simulink model "an_ch"  (Simulink 3.00)
settings: Solver=ode45  StartTime=0.0  StopTime=20  MaxStep=.01  RelTol=1e-3  AbsTol=1e-3
values from neighbouring files (symbols this model uses):
  den = 1    [ASS1_SIS.M]    (also in ASS_APPR.M; ASS_SIS.M; MYFBODE.M = b; MYNYQ.M = b)
  den_c = 1    [ASS1_SIS.M]    (also in ASS2_CN.M; ASS_C.M; ASS_SIS.M)
  num = 0    [ASS1_SIS.M]    (also in ASS_SIS.M; MYFBODE.M = a; MYNYQ.M = a; nyquistnew.m = a)
  num_c = 0    [ASS1_SIS.M]    (also in ASS2_CN.M; ASS_C.M; ASS_SIS.M)
  T = 0    [ASS1_SIS.M]    (also in ASS_APPR.M = 0; end; ASS_SIS.M; MYFBODE.M = rit)
undefined symbols (not defined in the file or in its folder): sfunyst
settings Model: SaveTime=off  SaveOutput=off  LastModifiedBy=Administrator

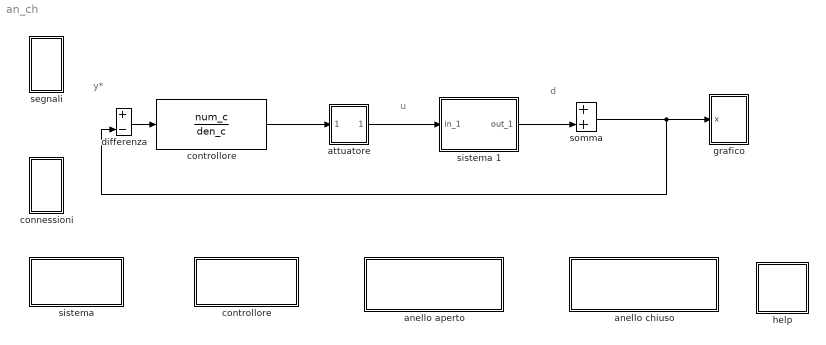
== system an_ch ==
  note: u
  note: d
  note: y*
  anello aperto : Subsystem
      mask Display: disp('analisi\n in anello aperto')
  anello chiuso : Subsystem
      mask Display: disp('analisi\n in anello chiuso')
  attuatore : Subsystem  mask{upperlimit=inf, lowerlimit=-inf}
      mask prompts: upperlimit "limite superiore"; lowerlimit "limite inferiore"
      mask Display: disp('A')
  connessioni : Subsystem
  controllore : Subsystem
      mask Display: disp('controllore')
  "controllore " : TransferFcn  Numerator=num_c  Denominator=den_c
      settings: OpenFcn=blocca
      mask Display: disp('controllore')
  differenza : Sum  Inputs=+-  SaturateOnIntegerOverflow=on
  grafico : Subsystem  mask(Storage scope.){@1=2, @2=-10, @3=10, @4=2000, @5='b-/r-/c-./w:/m*/ro/b+'}
      mask prompts: @1 "Initial Time Range:"; @2 "Initial y-min:"; @3 "Initial y-max:"; @4 "Storage pts.:"; @5 "Line type (rgbw-.:xo):"
      mask help:
      | Storage scope using MATLAB graph window.
      | Enter plotting ranges and line type.
      mask init:
      | npts = @4; color = @5; ax = [0, @1, @2, @3]; dt=-1;
      mask Help: This block uses a MATLAB figure window to plot the input signal.  The graph limits are automatically scaled to the min and max values of the signal stored in the scope's signal buffer.  Line type must be in quotes.  See the M-file sfunyst.m.
      mask Display: plot(0,0,100,100,[83,76,63,52,42,38,28,16,11,84,11,11,11,90,90,11],[75,58,47,54,72,80,84,74,65,65,65,90,40,40,90,90])
  help : Subsystem
      mask Display: disp('?')
  segnali : Subsystem
  sistema : Subsystem
      mask Display: disp('sistema')
  sistema 1 : Subsystem
      settings: OpenFcn=blocca
      mask Display: disp('sistema')
  "somma " : Sum  Inputs=++  SaturateOnIntegerOverflow=on
  wires:
  sistema 1/1(out_1) -> "somma "/2
  differenza/1 -> "controllore "/1
  "controllore "/1 -> attuatore/1(In1)
  attuatore/1(Out1) -> sistema 1/1(in_1)
  "somma "/1 -> grafico/1(x), differenza/2

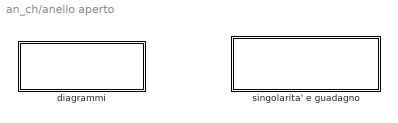
== system an_ch/anello aperto ==
  diagrammi : Subsystem
      mask Display: disp('diagrammi\n  \n (Bode e Nyquist)')
  singolarita' e guadagno : Subsystem
      settings: OpenFcn=sing_tot
      mask Type: singolarita' della f.d.t.
      mask Display: disp('singolarità,\n guadagno e ritardo')

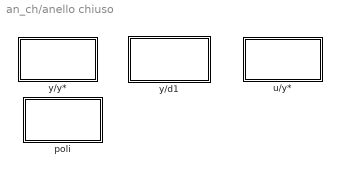
== system an_ch/anello chiuso ==
  poli : Subsystem
      settings: OpenFcn=sing_cl
      mask Type: singolarita' della f.d.t.
      mask Display: disp('poli')
  u/y* : Subsystem
      settings: OpenFcn=bodu_rif
      mask Display: disp('Bode u/y*')
  y/d1 : Subsystem
      settings: OpenFcn=bod2_d1
      mask Display: disp('Bode y/d')
  y/y* : Subsystem
      settings: OpenFcn=bod2_rif
      mask Display: disp('Bode y/y*')

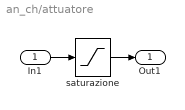
== system an_ch/attuatore ==
  In1 : Inport  Port=1  PortWidth=-1  SampleTime=-1  DataType=auto
      settings: SignalType=auto
  saturazione : Saturate  UpperLimit=upperlimit  LowerLimit=lowerlimit
  Out1 : Outport  Port=1
  wires:
  saturazione/1 -> Out1/1
  In1/1 -> saturazione/1

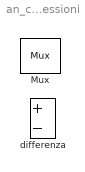
== system an_ch/connessioni ==
  Mux : Mux  Inputs=2
      settings: DisplayOption=none
  differenza : Sum  Inputs=+-  SaturateOnIntegerOverflow=on

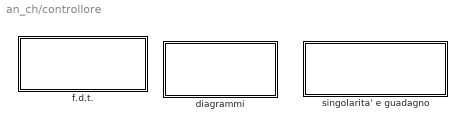
== system an_ch/controllore ==
  diagrammi : Subsystem
      mask Display: disp('diagrammi\n  \n (Bode e Nyquist)')
  f.d.t. : Subsystem
      settings: OpenFcn=ass_c
      mask Type: assegnamento controllore
      mask Display: disp('inserimento f.d.t.')
  singolarita' e guadagno : Subsystem
      settings: OpenFcn=sing_c
      mask Type: singolarita' della f.d.t.
      mask Display: disp('singolarità e guadagno')

== system an_ch/grafico ==
  x : Inport  Port=1  PortWidth=-1  SampleTime=-1  DataType=auto
      settings: SignalType=auto
  "S-function M-file which plots lines " : S-Function  LoadFcn=sfunyst([],[],[],'LoadBlock')  FunctionName=sfunyst  Parameters=ax, color, npts, dt  PortCounts=[]  SFunctionModules=''
      settings: CopyFcn=sfunyst([],[],[],'CopyBlock')  DeleteFcn=sfunyst([],[],[],'DeleteBlock')
  wires:
  x/1 -> "S-function M-file which plots lines "/1

== system an_ch/help ==
  note: i blocchi con l'ombreggiatura consentono
  note: - l'inserimento della funzione di trasferimento
  note: - l'ottenimento dei diagrammi di Bode e di Nyquist
  note: - la determinazione delle singolarità (poli e/o zeri) e/o del guadagno

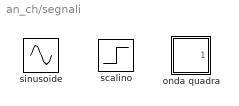
== system an_ch/segnali ==
  onda quadra : Subsystem  mask(Pulse Generator){@1=2, @2=1, @3=1, @4=0}
      mask prompts: @1 "Pulse period (secs):"; @2 "Pulse width:"; @3 "Pulse height:"; @4 "Pulse start time:"
      mask help: Pulse Generator.
      mask init:
      | Ts=@1; du=@2; ht=@3; stt=@4; ini=ones(length(ht),1); st1=rem(stt,Ts); st2=rem(stt+du,Ts);if(Ts<=1.2*du),ini=zeros(length(ht),1);end;
      mask Help: Pulse generator which ensures pulse\ntransitions are hit. Provides a vector of pulses when the height is entered as a vector.\nUnmask to see how it works.
      mask Display: plot(0,0,100,100,[90,75,75,60,60,35,35,20,20,10],[20,20,80,80,20,20,80,80,20,20])
  scalino : Step  Time=0  Before=0  After=1  SampleTime=-1
  sinusoide : Sin  Amplitude=1  Frequency=1  Phase=0  SampleTime=-1

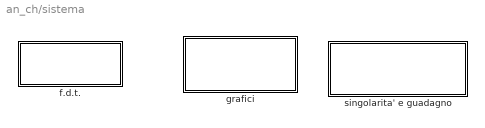
== system an_ch/sistema ==
  f.d.t. : Subsystem
      settings: OpenFcn=ass1_sis
      mask Type: assegnamento sistema
      mask Display: disp('inserimento\n f.d.t.')
  grafici : Subsystem
      mask Display: disp('grafici\n  \n (Bode e Nyquist)')
  singolarita' e guadagno : Subsystem
      settings: OpenFcn=sing_s
      mask Type: singolarita' della f.d.t.
      mask Display: disp('singolarità,\n guadagno e ritardo')

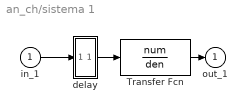
== system an_ch/sistema 1 ==
  in_1 : Inport  Port=1  PortWidth=-1  SampleTime=-1  DataType=auto
      settings: SignalType=auto
  Transfer Fcn : TransferFcn  Numerator=num  Denominator=den
  delay : Subsystem
  out_1 : Outport  Port=1
  wires:
  Transfer Fcn/1 -> out_1/1
  in_1/1 -> delay/1(in_1)
  delay/1(out_1) -> Transfer Fcn/1

== system an_ch/anello aperto/diagrammi ==
  Bode : Subsystem
      settings: OpenFcn=bode_tot
      mask Display: disp('Bode')
  Nyquist : Subsystem
      settings: OpenFcn=nyq_tot
      mask Display: disp('Nyquist')

== system an_ch/anello aperto/singolarita' e guadagno ==
  note: assegna

== system an_ch/anello chiuso/poli ==
  note: assegna

== system an_ch/anello chiuso/u/y* ==
  note: bode

== system an_ch/anello chiuso/y/d1 ==
  note: bode

== system an_ch/anello chiuso/y/y* ==
  note: bode

== system an_ch/controllore/diagrammi ==
  Subsystem1 : Subsystem
      settings: OpenFcn=nyq_c
      mask Display: disp('Nyquist')
  Subsystem2 : Subsystem
      settings: OpenFcn=bode_c
      mask Display: disp('Bode')

== system an_ch/controllore/f.d.t. ==
  note: assegna

== system an_ch/controllore/singolarita' e guadagno ==
  note: assegna

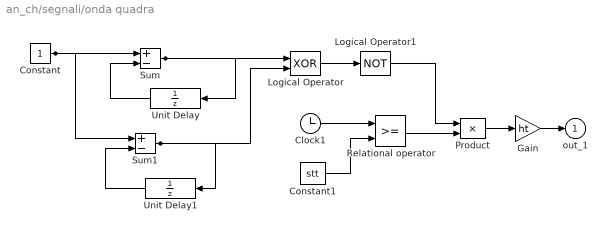
== system an_ch/segnali/onda quadra ==
  Clock1 : Clock
      settings: DisplayTime=off  Decimation=10
  Constant : Constant  Value=1
  Constant1 : Constant  Value=stt
  Gain : Gain  Gain=ht  SaturateOnIntegerOverflow=on
  Logical Operator : Logic  Operator=XOR  Inputs=2
  Logical Operator1 : Logic  Operator=NOT  Inputs=1
  Product : Product  Inputs=2  SaturateOnIntegerOverflow=on
  Relational operator : RelationalOperator  Operator=>=
  Sum : Sum  Inputs=+-  SaturateOnIntegerOverflow=on
  Sum1 : Sum  Inputs=+-  SaturateOnIntegerOverflow=on
  Unit Delay : UnitDelay  Orientation=left  X0=0  SampleTime=[Ts,st1]
  Unit Delay1 : UnitDelay  Orientation=left  X0=ini  SampleTime=[Ts,st2]
  out_1 : Outport  Port=1
  wires:
  Logical Operator1/1 -> Product/1
  Logical Operator/1 -> Logical Operator1/1
  Constant1/1 -> Relational operator/2
  Gain/1 -> out_1/1
  Product/1 -> Gain/1
  Relational operator/1 -> Product/2
  Clock1/1 -> Relational operator/1
  Unit Delay/1 -> Sum/2
  Unit Delay1/1 -> Sum1/2
  Constant/1 -> Sum/1, Sum1/1
  Sum/1 -> Unit Delay/1, Logical Operator/1
  Sum1/1 -> Unit Delay1/1, Logical Operator/2

== system an_ch/sistema/f.d.t. ==
  note: assegna

== system an_ch/sistema/grafici ==
  Subsystem1 : Subsystem
      settings: OpenFcn=nyq_sis
      mask Display: disp('Nyquist')
  Subsystem2 : Subsystem
      settings: OpenFcn=bode_sis
      mask Display: disp('Bode')

== system an_ch/sistema/singolarita' e guadagno ==
  note: assegna

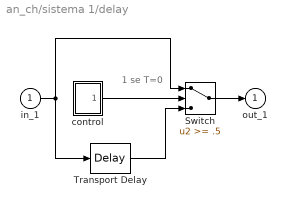
== system an_ch/sistema 1/delay ==
  note: 1 se T=0
  in_1 : Inport  Port=1  PortWidth=-1  SampleTime=-1  DataType=auto
      settings: SignalType=auto
  Switch : Switch  Threshold=.5
  Transport Delay : TransportDelay  DelayTime=T  InitialInput=0  BufferSize=1024
  control : Subsystem
  out_1 : Outport  Port=1
  wires:
  Transport Delay/1 -> Switch/3
  in_1/1 -> Switch/1, Transport Delay/1
  Switch/1 -> out_1/1
  control/1(out_1) -> Switch/2

== system an_ch/anello aperto/diagrammi/Bode ==
  note: bode

== system an_ch/anello aperto/diagrammi/Nyquist ==
  note: bode

== system an_ch/controllore/diagrammi/Subsystem1 ==
  note: bode

== system an_ch/controllore/diagrammi/Subsystem2 ==
  note: bode

== system an_ch/sistema/grafici/Subsystem1 ==
  note: bode

== system an_ch/sistema/grafici/Subsystem2 ==
  note: bode

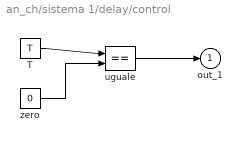
== system an_ch/sistema 1/delay/control ==
  T : Constant  Value=T
  uguale : RelationalOperator  Operator===
  zero : Constant  Value=0
  out_1 : Outport  Port=1
  wires:
  zero/1 -> uguale/2
  T/1 -> uguale/1
  uguale/1 -> out_1/1
